simulink model "mask"  (R2020a)
settings: Solver=VariableStepAuto  StartTime=0.0  StopTime=10.0  RelTol=1e-3
model workspace (MAT data in the model file):
  A = 10
  B = 20
libraries: PI_lib x2
settings Model: Creator=sonal  LastModifiedBy=sonal

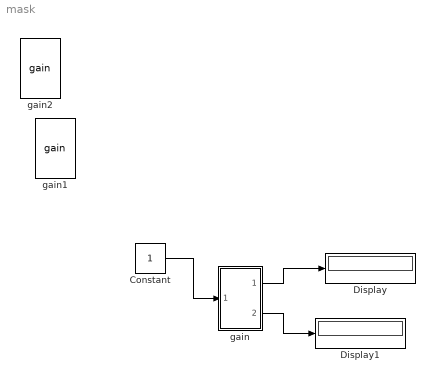
== system mask ==
  Constant : Constant
  Display : Display
  Display1 : Display
  gain : Subsystem  mask{A=1, B=2}
      mask Display: image('ic.jpg'); % Use "Edit Image" on toolstrip to change.
  gain1 : PI_lib/gain  A=1  B=2
  gain2 : PI_lib/gain  A=1  B=2
  wires:
  Constant/1 -> gain/1(In1)
  gain/1(Out1) -> Display/1
  gain/2(Out2) -> Display1/1

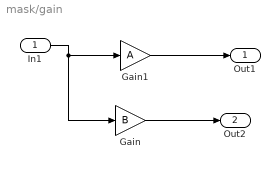
== system mask/gain ==
  In1 : Inport
  Gain : Gain  Gain=B
  Gain1 : Gain  Gain=A
  Out1 : Outport
  Out2 : Outport  Port=2
  wires:
  In1/1 -> Gain/1, Gain1/1
  Gain/1 -> Out2/1
  Gain1/1 -> Out1/1
